simulink model "rocket_simulation"  (R2025a)
settings: Solver=VariableStepAuto  StartTime=0.0  StopTime=60  RelTol=1e-3
values from neighbouring files (symbols this model uses):
  thrust = [471.175 1413.524 2180.151 2224.366 2190.483 2156.6 2124.312 2117.203 2118.781 2120.36 2121.938 2123.517 ... (112 elements, 112x1)]    [thrust_profile.mat]
undefined symbols (not defined in the file or in its folder): F, Light, MIL
libraries: aerolibwind2 x1, aerolibbdyn x1, aerolibatmos2 x1

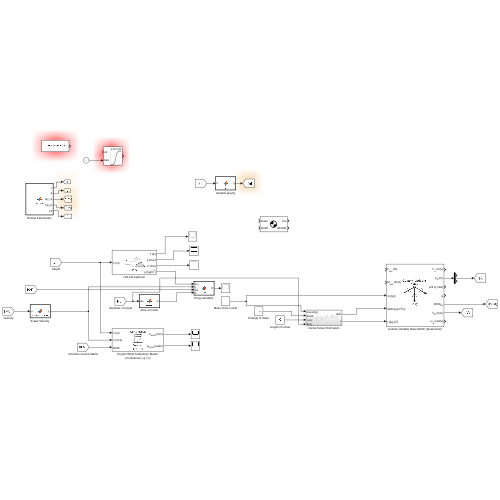
[thumbnail: Simulink's stored preview of the top-level diagram]
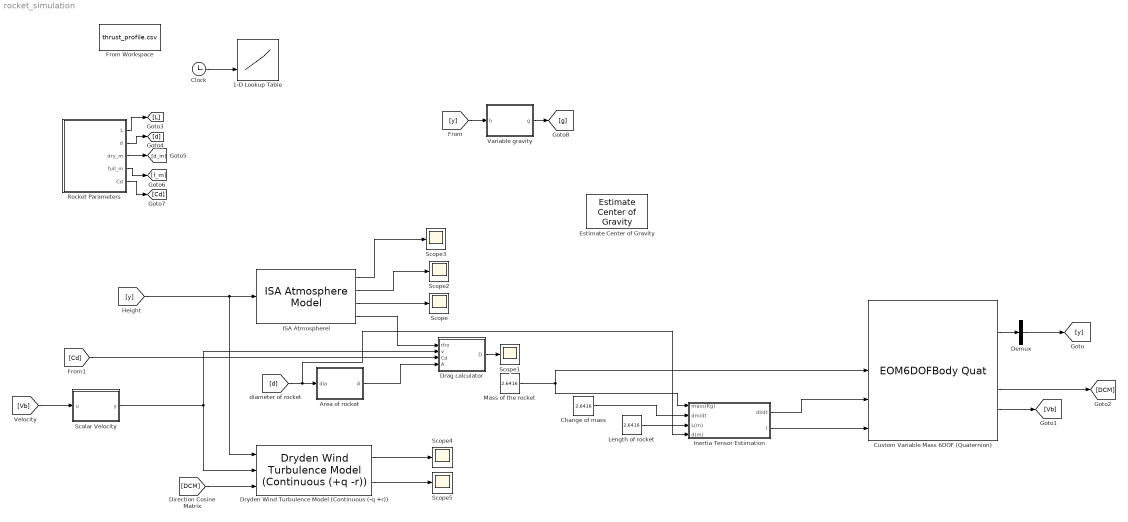
== system rocket_simulation ==
  1-D Lookup Table : Lookup_n-D  NumberOfTableDimensions=1  BreakpointsForDimension1Source=Input port  BreakpointsForDimension1=[-5:5]  Table=thrust  InternalRulePriority=Speed  RndMeth=Simplest
      settings: InputPortMap=u0,p5
  Area of rocket : MATLAB Function  TreatAsAtomicUnit=on
  Change of mass : Constant  Value=2.6416
  Clock : Clock
  Custom Variable Mass 6DOF (Quaternion) : EOM6DOFBodyQuat  mtype=Custom Variable
  Demux : Demux  Outputs=3
  Drag calculator : MATLAB Function  TreatAsAtomicUnit=on
  Dryden Wind Turbulence Model (Continuous (-q +r)) : aerolibwind2/Dryden Wind Turbulence Model  (Continuous (+q -r))  units=Metric (MKS)  spec=MIL-F-8785C  model=Continuous Dryden (-q +r)  W20=15  Wdeg=0  TurbProb=10^-2 - Light  L_high=533.4  Wingspan=10  ts=0.1  Seed=[23341 23342 23343 23344]  T_on=on
      settings: LibrarySourceBlock=|
      | aerolibwind2/Dryden Wind Turbulence Model
      | (Continuous (-q +r))
  Estimate Center of Gravity : aerolibbdyn/Estimate Center of Gravity  fmass=2  emass=1  fcg=[1 1 1]'  ecg=[0.5 0.5 0.5]'
  From Workspace : FromWorkspace  VariableName=thrust_profile.csv
  ISA Atmospherel : aerolibatmos2/ISA Atmosphere Model  useExtended=off  action=None  custom=off  viscosityOut=off  g=9.80665  gamma=1.4  R=287.0531  L=0.0065  h_trop=11000  h_strat=20000  rho0=1.225  P0=101325  T0=288.15  h0=0  S=110.4  Tref=273.15  muref=1.716e-5
  Inertia Tensor Estimation : Subsystem
  Length of rocket : Constant  Value=2.6416
  Mass of the rocket : Constant  Value=2.6416
  Rocket Parameters : MATLAB Function  TreatAsAtomicUnit=on
  "Scalar Velocity " : MATLAB Function  TreatAsAtomicUnit=on
  Scope{,1..5} (6 alike) : Scope
      Scope settings: ActiveDisplayYMinimum=101189.91706788937  ActiveDisplayYMaximum=101340.00921467897
      Scope1 settings: ActiveDisplayYMinimum=101189.91706788937  ActiveDisplayYMaximum=101340.00921467897
      Scope2 settings: ActiveDisplayYMinimum=340.25094300687613  ActiveDisplayYMaximum=340.29892228332653  DataLoggingVariableName=ScopeData2
      Scope3 settings: ActiveDisplayYMinimum=288.076875  ActiveDisplayYMaximum=288.158125  DataLoggingVariableName=ScopeData3
      Scope4 settings: ActiveDisplayYMinimum=-5.0798651721078141  ActiveDisplayYMaximum=6.2761631966690334  DataLoggingVariableName=ScopeData4
      Scope5 settings: ActiveDisplayYMinimum=-0.4513348332530695  ActiveDisplayYMaximum=0.50877727433739572  DataLoggingVariableName=ScopeData5
  Variable gravity : MATLAB Function  TreatAsAtomicUnit=on
  wires:
  [y] -> ISA Atmospherel/1, Dryden Wind Turbulence Model (Continuous (-q +r))/1
  ISA Atmospherel/4 -> Drag calculator/1(rho)
  ISA Atmospherel/3 -> Scope/1
  ISA Atmospherel/2 -> Scope2/1
  ISA Atmospherel/1 -> Scope3/1
  [DCM] -> Dryden Wind Turbulence Model (Continuous (-q +r))/3
  "Scalar Velocity "/1(y) -> Drag calculator/2(v), Dryden Wind Turbulence Model (Continuous (-q +r))/2
  [Cd] -> Drag calculator/3(Cd)
  Drag calculator/1(D) -> Scope1/1
  Dryden Wind Turbulence Model (Continuous (-q +r))/1 -> Scope4/1
  Dryden Wind Turbulence Model (Continuous (-q +r))/2 -> Scope5/1
  [d] -> Inertia Tensor Estimation/4(d(m)), Area of rocket/1(dia)
  Area of rocket/1(A) -> Drag calculator/4(A)
  Inertia Tensor Estimation/1(dI/dt) -> Custom Variable Mass 6DOF (Quaternion)/4
  Inertia Tensor Estimation/2(I) -> Custom Variable Mass 6DOF (Quaternion)/5
  Mass of the rocket/1 -> Custom Variable Mass 6DOF (Quaternion)/3, Inertia Tensor Estimation/1(mass(Kg))
  Change of mass/1 -> Inertia Tensor Estimation/2(dm/dt)
  Length of rocket/1 -> Inertia Tensor Estimation/3(L(m))
  Custom Variable Mass 6DOF (Quaternion)/2 -> Demux/1
  Demux/2 -> [y]
  Custom Variable Mass 6DOF (Quaternion)/6 -> [Vb]
  [Vb] -> "Scalar Velocity "/1(u)
  Custom Variable Mass 6DOF (Quaternion)/5 -> [DCM]
  Rocket Parameters/1(L) -> [L]
  Rocket Parameters/2(d) -> [d]
  Rocket Parameters/4(full_m) -> [f_m]
  Rocket Parameters/3(dry_m) -> [d_m]
  Rocket Parameters/5(Cd) -> [Cd]
  [y] -> Variable gravity/1(h)
  Variable gravity/1(g) -> [g]
  Clock/1 -> 1-D Lookup Table/2

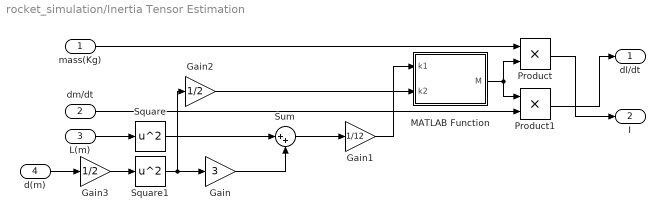
== system rocket_simulation/Inertia Tensor Estimation ==
  mass(Kg) : Inport
  dm/dt : Inport  Port=2
  L(m) : Inport  Port=3
  d(m) : Inport  Port=4
  Gain : Gain  Gain=3
  Gain1 : Gain  Gain=1/12
  Gain2 : Gain  Gain=1/2
  Gain3 : Gain  Gain=1/2
  MATLAB Function : MATLAB Function  TreatAsAtomicUnit=on
  Product : Product
  Product1 : Product
  Square : Math  Operator=square
  Square1 : Math  Operator=square
  Sum : Sum  Inputs=|++
  dI/dt : Outport
  I : Outport  Port=2
  wires:
  L(m)/1 -> Square/1
  Square1/1 -> Gain2/1, Gain/1
  Square/1 -> Sum/1
  Gain/1 -> Sum/2
  Sum/1 -> Gain1/1
  Gain1/1 -> MATLAB Function/1(k1)
  Gain2/1 -> MATLAB Function/2(k2)
  MATLAB Function/1(M) -> Product1/1, Product/2
  mass(Kg)/1 -> Product/1
  dm/dt/1 -> Product1/2
  Product1/1 -> dI/dt/1
  Product/1 -> I/1
  Gain3/1 -> Square1/1
  d(m)/1 -> Gain3/1

== matlab function rocket_simulation/Scalar Velocity  ==
  data: u input; y output
function y = magnitude(u)
    y = norm(u);

== matlab function rocket_simulation/Drag calculator ==
  data: rho input; D output; v input; Cd input; A input
function D = drag(rho, v, Cd, A)
    D = 0.5 * rho * v^2 * Cd * A;

== matlab function rocket_simulation/Area of rocket ==
  data: dia input; A output
function A = area(dia)
    A = pi*((dia)^2)/4;

== matlab function rocket_simulation/Inertia Tensor Estimation/MATLAB Function ==
  data: k1 input; M output; k2 input
function M =diag_mat(k1, k2)
    M = diag([k1,k1,k2]);

== matlab function rocket_simulation/Variable gravity ==
  data: h input; g output
function g = g(h)
    % h is altitude in meters
    R = 6.371e6;          % Earth radius in meters
    g0 = 9.80665;         % Standard gravity in m/s^2
    g = g0 * (R / (R + h))^2;

== matlab function rocket_simulation/Rocket Parameters ==
  data: L output; d output; dry_m output; full_m output; Cd output
function [L, d, dry_m, full_m, Cd] = param()
    L = 2.6416; % Length in meters (104 in)
    d = 0.1524; % Diameter in meters (6 in)
    dry_m = 17.190; % mass in Kg
    full_m = 23.872; % mass in Kg
    Cd = 1; % Drag coefficient unitless
